simulink model "ModelCL"  (R2021a)
settings: Solver=VariableStepAuto  StartTime=0.0  StopTime=10.0  RelTol=1e-3
values from neighbouring files (symbols this model uses):
  K1 = Ka(:,1:12)    [testCtr.m]
  Ki = -Ka(:,13:16)    [testCtr.m]
undefined symbols (not defined in the file or in its folder): C, g0, M
libraries: shared6dof x1
settings Model: Creator=Adam  LastModifiedBy=Adam

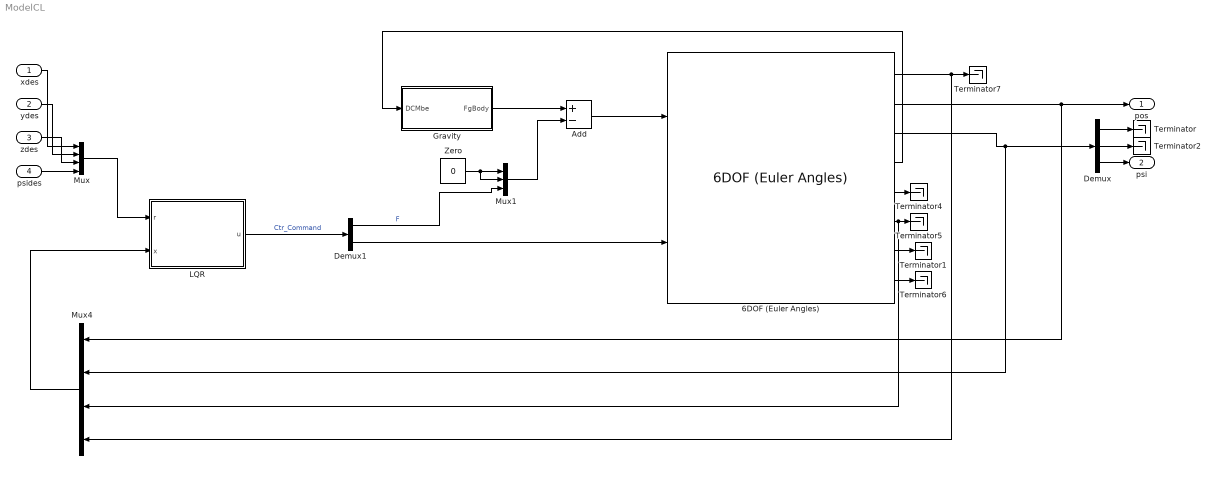
== system ModelCL ==
  xdes : Inport
  ydes : Inport  Port=2
  zdes : Inport  Port=3
  psides : Inport  Port=4
  6DOF (Euler Angles) : shared6dof/6DOF (Euler Angles)  units=Metric (MKS)  mtype=Fixed  rep=Euler Angles  xme_0=x0  Vm_0=[0 0 0]  eul_0=[0 0 0]  pm_0=[0 0 0]  mass_0=M  mass_e=0.5  mass_f=2.0  inertia=Ib  inertia_e=eye(3)  inertia_f=2*eye(3)  k_quat=1.0  vre_flag=on  abi_flag=off  aMode=0  xme_statename='Xe'  Vm_statename='Ve'  eul_statename='Euler'  quat_statename=''  pm_statename='Omega'  mass_statename=''
      settings: SourceProductBaseCode=AE,PW,DR,MT,UV,VE
  Add : Sum  Inputs=+-
  Demux : Demux  Outputs=3
  Demux1 : Demux  Outputs=2
  "Gravity " : Subsystem
  LQR : Subsystem
  Mux : Mux
  Mux1 : Mux  Inputs=3
  Mux4 : Mux
  Terminator{,1..2,4..7} (7 alike) : Terminator
  Zero : Constant  Value=0  OutDataTypeStr=Inherit: Inherit via back propagation
  pos : Outport
  psi : Outport  Port=2
  wires:
  6DOF (Euler Angles)/7 -> Terminator1/1
  Zero/1 -> Mux1/2, Mux1/1
  "Gravity "/1(FgBody) -> Add/1
  6DOF (Euler Angles)/4 -> "Gravity "/1(DCMbe)
  Mux1/1 -> Add/2
  Add/1 -> 6DOF (Euler Angles)/1
  Demux/1 -> Terminator/1
  Demux/2 -> Terminator2/1
  Demux/3 -> psi/1
  6DOF (Euler Angles)/5 -> Terminator4/1
  6DOF (Euler Angles)/8 -> Terminator6/1
  Demux1/2 -> 6DOF (Euler Angles)/2
  6DOF (Euler Angles)/6 -> Mux4/3, Terminator5/1
  Demux1/1 -> Mux1/3  "F"
  6DOF (Euler Angles)/2 -> Mux4/1, pos/1
  6DOF (Euler Angles)/1 -> Mux4/4, Terminator7/1
  Mux4/1 -> LQR/2(x)
  LQR/1(u) -> Demux1/1  "Ctr_Command"
  6DOF (Euler Angles)/3 -> Mux4/2, Demux/1
  psides/1 -> Mux/4
  Mux/1 -> LQR/1(r)
  zdes/1 -> Mux/3
  ydes/1 -> Mux/2
  xdes/1 -> Mux/1

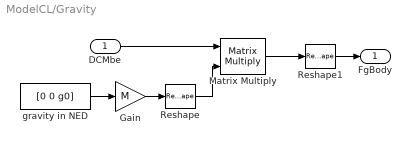
== system ModelCL/Gravity  ==
  DCMbe : Inport
  Gain : Gain  Gain=M
  Matrix Multiply : Product  Multiplication=Matrix(*)
  Reshape : Reshape  OutputDimensionality=Column vector (2-D)
  Reshape1 : Reshape
  gravity in NED : Constant  Value=[0 0 g0]
  FgBody : Outport
  wires:
  gravity in NED/1 -> Gain/1
  Reshape/1 -> Matrix Multiply/2
  Matrix Multiply/1 -> Reshape1/1
  DCMbe/1 -> Matrix Multiply/1
  Gain/1 -> Reshape/1
  Reshape1/1 -> FgBody/1

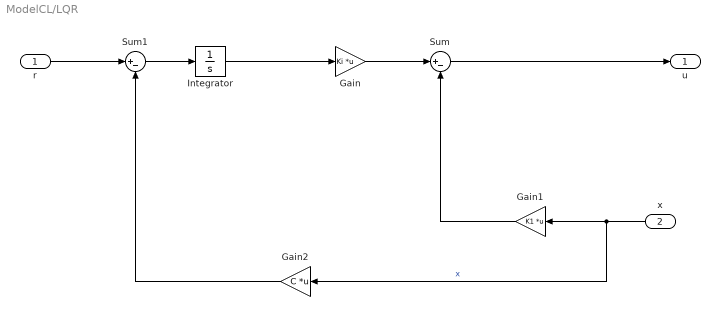
== system ModelCL/LQR ==
  r : Inport
  x : Inport  Port=2
  Gain : Gain  Gain=Ki  Multiplication=Matrix(K*u)
  Gain1 : Gain  Gain=K1  Multiplication=Matrix(K*u)
  Gain2 : Gain  Gain=C  Multiplication=Matrix(K*u)
  Integrator : Integrator
  Sum : Sum  Inputs=|+-
  Sum1 : Sum  Inputs=|+-
  u : Outport
  wires:
  Sum/1 -> u/1
  Gain2/1 -> Sum1/2
  r/1 -> Sum1/1
  Gain/1 -> Sum/1
  Sum1/1 -> Integrator/1
  x/1 -> Gain1/1, Gain2/1  "x"
  Gain1/1 -> Sum/2
  Integrator/1 -> Gain/1
